simulink model "part2_Power_Bandwidth_SNR"  (R2024a)
settings: Solver=VariableStepAuto  StartTime=0.0  StopTime=10.0  RelTol=1e-3
libraries: dspstat3 x3, dspmathops x3, dspfdesign x2, dspsrcs4 x1, simulink x1, spsTriangleGeneratorLib x1
settings Model: Creator=alice  LastModifiedBy=alice

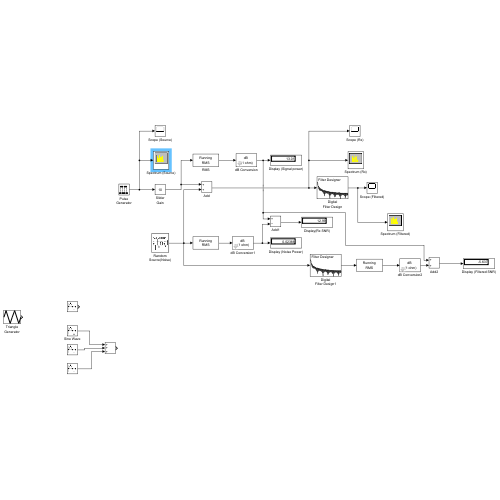
[thumbnail: Simulink's stored preview of the top-level diagram]
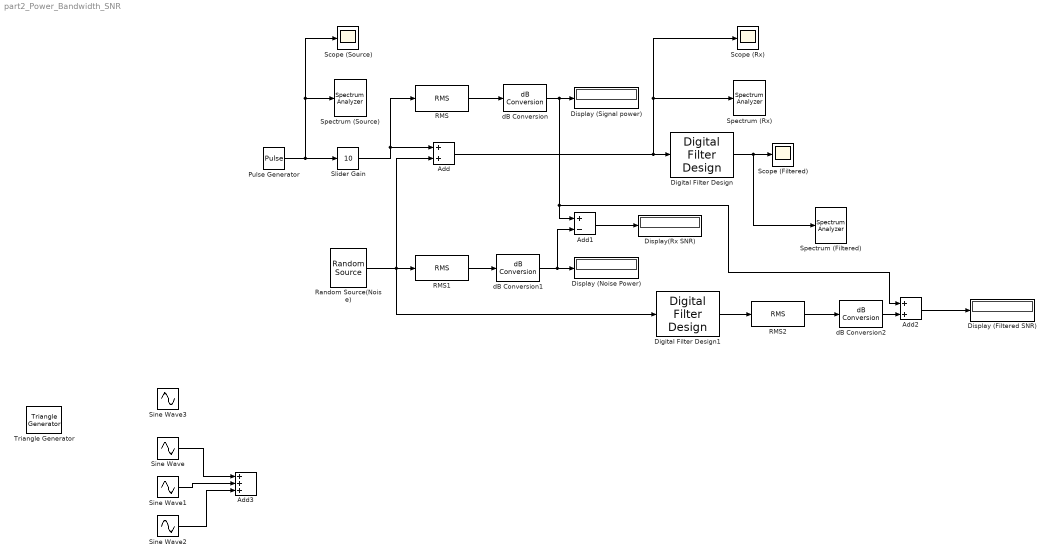
== system part2_Power_Bandwidth_SNR ==
  Add : Sum
  Add1 : Sum  Inputs=+-
  Add2 : Sum
  Add3 : Sum  Inputs=+++
  Digital Filter Design : dspfdesign/Digital Filter Design  mwdsp_browser_bugfix_var=off
  Digital Filter Design1 : dspfdesign/Digital Filter Design  mwdsp_browser_bugfix_var=off
  Display (Filtered SNR) : Display
  Display (Noise Power) : Display
  Display (Signal power) : Display
  Display(Rx SNR) : Display
  Pulse Generator : DiscretePulseGenerator  Period=5000  PulseWidth=1000  SampleTime=1e-4
  RMS : dspstat3/RMS  run=on  directionMode=Each column  dimension=1  InputProcessing=Columns as channels (frame based)  reset_popup=None
  RMS1 : dspstat3/RMS  run=on  directionMode=Each column  dimension=1  InputProcessing=Columns as channels (frame based)  reset_popup=None
  RMS2 : dspstat3/RMS  run=on  directionMode=Each column  dimension=1  InputProcessing=Columns as channels (frame based)  reset_popup=None
  Random Source(Noise) : dspsrcs4/Random Source  SrcType=Gaussian  MinVal=0  MaxVal=1  MeanVal=0  VarVal=1  RepMode=Specify seed  rawSeed=1  IsInherit=off  SampTime=1e-4  SampFrame=1  OutComplex=Real  DataType=double  SimulateUsing=Interpreted execution
  Scope (Filtered) : Scope
  Scope (Rx) : Scope
  Scope (Source) : Scope
  Sine Wave : Sin  SineType=Sample based  Amplitude=0.5  Samples=1000  SampleTime=1e-4
  Sine Wave1 : Sin  SineType=Sample based  Amplitude=2  Samples=500  SampleTime=1e-4
  Sine Wave2 : Sin  SineType=Sample based  Amplitude=1.5  Samples=100  SampleTime=1e-4
  Sine Wave3 : Sin  SineType=Sample based  Samples=100  SampleTime=1e-4
  Slider Gain : simulink/Math Operations/Slider Gain  gain=10  low=0  high=10
  Spectrum (Filtered) : SpectrumAnalyzer  WindowPosition=[229.000000,167.000000,800.000000,500.000000,]  ScopeFrameLocation=window  YLimits=[-25.82014179,57.92164035]
  Spectrum (Rx) : SpectrumAnalyzer  WindowPosition=[240.000000,150.000000,800.000000,500.000000,]  ScopeFrameLocation=window  YLimits=[-14.02574207,49.38874797]  SelectedToolstripTab=spectrumAnalyzerToolstrip.measurementsTab
  Spectrum (Source) : SpectrumAnalyzer  WindowPosition=[1.000000,49.000000,1280.000000,729.000000,]  ScopeFrameLocation=window  RBWSource=Property  RBW=3  YLimits=[-55.28859429,28.04167515]  SelectedToolstripTab=spectrumAnalyzerToolstrip.estimationTab
  Triangle Generator : spsTriangleGeneratorLib/Triangle Generator  Freq=5  Phase=90  Ts=1e-4
  dB Conversion : dspmathops/dB Conversion  dBtype=dB  intype=Amplitude  R=1  fuzz=off
  dB Conversion1 : dspmathops/dB Conversion  dBtype=dB  intype=Amplitude  R=1  fuzz=off
  dB Conversion2 : dspmathops/dB Conversion  dBtype=dB  intype=Amplitude  R=1  fuzz=off
  wires:
  Pulse Generator/1 -> Scope (Source)/1, Spectrum (Source)/1, Slider Gain/1
  Slider Gain/1 -> Add/1, RMS/1
  Random Source(Noise)/1 -> Digital Filter Design1/1, Add/2, RMS1/1
  RMS1/1 -> dB Conversion1/1
  RMS/1 -> dB Conversion/1
  dB Conversion1/1 -> Add1/2, Display (Noise Power)/1
  Add1/1 -> Display(Rx SNR)/1
  Add/1 -> Spectrum (Rx)/1, Scope (Rx)/1, Digital Filter Design/1
  Digital Filter Design/1 -> Spectrum (Filtered)/1, Scope (Filtered)/1
  Digital Filter Design1/1 -> RMS2/1
  RMS2/1 -> dB Conversion2/1
  dB Conversion2/1 -> Add2/2
  dB Conversion/1 -> Add2/1, Add1/1, Display (Signal power)/1
  Add2/1 -> Display (Filtered SNR)/1
  Sine Wave/1 -> Add3/1
  Sine Wave1/1 -> Add3/2
  Sine Wave2/1 -> Add3/3
